simulink model "ATRIAS_vnmc"  (R2015a)
settings: Solver=ode45  StartTime=0.0  StopTime=60  FixedStep=1e-3  MinStep=1e-6  RelTol=1e-3  AbsTol=1e-4
values from neighbouring files (symbols this model uses):
  initial_boom_yaw = initial_boom_yaw + delta_yaw0    [run_model.m]
  max_floor_diff = cost_fun_opts.max_floor_diff    [opt_cmaes.m]    (also in run_model.m; set_all_params_simple.m = 0)
  noise_on_off = cost_fun_opts.noise_on_off    [opt_cmaes.m]    (also in run_model.m; set_all_params_simple.m = 0)
  noise_seed = cost_fun_opts.noise_seed    [opt_cmaes.m]    (also in run_model.m; set_all_params_simple.m = 1)
  noise_variance = cost_fun_opts.noise_variance    [opt_cmaes.m]    (also in run_model.m; set_all_params_simple.m = 0.000174532925199)
  SEA_swing_ctrl_on_off = cost_fun_opts.SEA_swing_ctrl_on_off    [opt_cmaes.m]    (also in run_model.m; set_all_params_simple.m = 0)
  sim_t = simout.twalk    [run_model.m]
  steady_dist = cost_fun_opts.steady_dist    [opt_cmaes.m]    (also in run_model.m; set_all_params_simple.m = 10)
  ts_anim = 0.0333    [run_model.m]
undefined symbols (not defined in the file or in its folder): A1_notch_f1, A2_notch_f1, A_lpf_dtau, A_lpf_velocity, B1_lpf_dtau, B1_lpf_velocity, B1_notch_f1, B2_lpf_dtau, B2_lpf_velocity, B2_notch_f1, b_hmotor, b_leg_spring, b_rotor, base_color_d, boom_color_d, boom_mount_to_center_diagonal, breakaway_friction, c, c_jointstop, com_height_offset, contactThr, coulomb_friction, CtrlPar_theta0, D12_S, D12_T, d_com, ddx_max, ddy_max, delta_phi_max, delta_phi_max_buffer, delta_phi_max_dropoff, delta_phi_min, des_forward_velocity, DS_width, dtau_des_max, dtheta0_vmc, dx0_vmc, dy_max, eref, fblink_color_d, fcut_acceleration, floor_color_d, floor_tile_width, floor_zero_height, FmaxBFSH, FmaxGLU, FmaxHAM, FmaxHFL, FmaxRF, FmaxVAS, FPCtrlPar, friction_linear_zone, g, gain_nodes_sea_torque, gamma_stance_thr, gamma_swing_thr, hip_height, HIP_MTR_MAX_CONT_TORQUE, HIP_MTR_MAX_TORQUE, hshaft_color_d ... (+236)
libraries: sm_lib x280, nesl_utility x174, simulink x114, simulink_extras x58, fl_lib x16, mblibv1 x2, dspswit3 x2
(part 8 of 23)

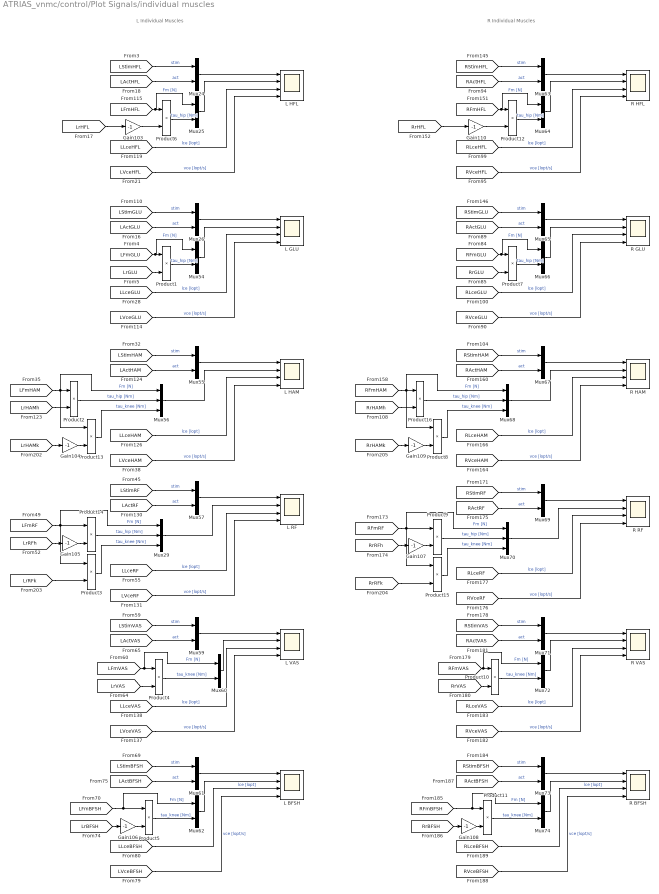
== system ATRIAS_vnmc/control/Plot Signals/individual muscles ==
  note: L Individual Muscles
  note: R Individual Muscles
  Gain{103..110} (8 alike) : Gain  Gain=-1
  L BFSH : Scope  NumInputPorts=4
      settings: ShowLegends=on  TimeRange=1  YMin=5.55112e-17~-50~0.65~-15  YMax=1~300~1~15  SaveName=ScopeData33
  L GLU : Scope  NumInputPorts=4
      settings: ShowLegends=on  TimeRange=1  YMin=0~0~0.4~-20  YMax=1~260.2739726027394~1~20  SaveName=ScopeData37
  L HAM : Scope  NumInputPorts=4
      settings: ShowLegends=on  TimeRange=1  YMin=0~-175.6756756756768~0.6000000000000001~-20  YMax=1~716.2162162162167~1~20  SaveName=ScopeData39
  L HFL : Scope  NumInputPorts=4
      settings: ShowLegends=on  TimeRange=1  YMin=0~-315.0684931506839~0.8~-20  YMax=1~424.6575342465767~1.4~20  SaveName=ScopeData41
  L RF : Scope  NumInputPorts=4
      settings: ShowLegends=on  TimeRange=1  YMin=0~-119.8630136986303~0.7000000000000001~-20  YMax=1~147.2602739726026~1~20  SaveName=ScopeData44
  L VAS : Scope  NumInputPorts=4
      settings: ShowLegends=on  TimeRange=2.5  YMin=0~0~0.5~-20  YMax=1~6000~1.5~20  SaveName=ScopeData47
  Mux{24..26,54..55,57,59..67,69,71..74} (20 alike) : Mux  Inputs=2
  Mux{29,56,68,70} (4 alike) : Mux  Inputs=3
  Product{1..16} (16 alike) : Product  RndMeth=Zero
  R BFSH : Scope  NumInputPorts=4
      settings: ShowLegends=on  TimeRange=1.6  YMin=130~-300~-5~-5  YMax=200~300~5~5  SaveName=ScopeData58
  R GLU : Scope  NumInputPorts=4
      settings: ShowLegends=on  TimeRange=1.6  YMin=130~-300~-5~-5  YMax=200~300~5~5  SaveName=ScopeData60
  R HAM : Scope  NumInputPorts=4
      settings: ShowLegends=on  TimeRange=1.6  YMin=130~-300~-5~-5  YMax=200~300~5~5  SaveName=ScopeData62
  R HFL : Scope  NumInputPorts=4
      settings: ShowLegends=on  TimeRange=1.6  YMin=130~-300~-5~-5  YMax=200~300~5~5  SaveName=ScopeData64
  R RF : Scope  NumInputPorts=4
      settings: ShowLegends=on  TimeRange=1.6  YMin=130~-300~-5~-5  YMax=200~300~5~5  SaveName=ScopeData67
  R VAS : Scope  NumInputPorts=4
      settings: ShowLegends=on  TimeRange=1.6  YMin=130~-300~-5~-5  YMax=200~300~5~5  SaveName=ScopeData70
  wires:
  [LStimHFL] -> Mux24/1  "stim"
  [LFmHFL] -> Mux25/1, Product6/1  "Fm [N]"
  [LrHFL] -> Gain103/1
  Product6/1 -> Mux25/2  "tau_hip [Nm]"
  [LActHFL] -> Mux24/2  "act"
  Mux24/1 -> L HFL/1
  Mux25/1 -> L HFL/2
  [LLceHFL] -> L HFL/3  "lce [lopt]"
  [LVceHFL] -> L HFL/4  "vce [lopt/s]"
  [LStimGLU] -> Mux26/1  "stim"
  [LFmGLU] -> Mux54/1, Product1/1  "Fm [N]"
  [LrGLU] -> Product1/2
  Product1/1 -> Mux54/2  "tau_hip [Nm]"
  [LActGLU] -> Mux26/2  "act"
  Mux26/1 -> L GLU/1
  Mux54/1 -> L GLU/2
  [LLceGLU] -> L GLU/3  "lce [lopt]"
  [LVceGLU] -> L GLU/4  "vce [lopt/s]"
  [LStimHAM] -> Mux55/1  "stim"
  [LFmHAM] -> Product2/1, Product13/1, Mux56/1  "Fm [N]"
  [LrHAMh] -> Product2/2
  Product2/1 -> Mux56/2  "tau_hip [Nm]"
  [LActHAM] -> Mux55/2  "act"
  Mux55/1 -> L HAM/1
  Mux56/1 -> L HAM/2
  [LLceHAM] -> L HAM/3  "lce [lopt]"
  [LVceHAM] -> L HAM/4  "vce [lopt/s]"
  [LStimRF] -> Mux57/1  "stim"
  [LActRF] -> Mux57/2  "act"
  Mux57/1 -> L RF/1
  [LLceRF] -> L RF/3  "lce [lopt]"
  [LVceRF] -> L RF/4  "vce [lopt/s]"
  [LStimVAS] -> Mux59/1  "stim"
  [LFmVAS] -> Product4/1, Mux60/1  "Fm [N]"
  Product4/1 -> Mux60/2  "tau_knee [Nm]"
  [LActVAS] -> Mux59/2  "act"
  Mux59/1 -> L VAS/1
  Mux60/1 -> L VAS/2
  [LLceVAS] -> L VAS/3  "lce [lopt]"
  [LVceVAS] -> L VAS/4  "vce [lopt/s]"
  [LStimBFSH] -> Mux61/1  "stim"
  [LFmBFSH] -> Mux62/1, Product5/1  "Fm [N]"
  [LrBFSH] -> Gain106/1
  Product5/1 -> Mux62/2  "tau_knee [Nm]"
  [LActBFSH] -> Mux61/2  "act"
  Mux61/1 -> L BFSH/1
  Mux62/1 -> L BFSH/2
  [LLceBFSH] -> L BFSH/3  "lce [lopt]"
  [LVceBFSH] -> L BFSH/4  "vce [lopt/s]"
  Gain103/1 -> Product6/2
  [LrHAMk] -> Gain104/1
  Product13/1 -> Mux56/3  "tau_knee [Nm]"
  [LFmRF] -> Product14/1, Product3/1, Mux29/1  "Fm [N]"
  [LrRFh] -> Gain105/1
  Product14/1 -> Mux29/2  "tau_hip [Nm]"
  [LrRFk] -> Product3/2
  Product3/1 -> Mux29/3  "tau_knee [Nm]"
  Gain105/1 -> Product14/2
  Mux29/1 -> L RF/2
  [LrVAS] -> Product4/2
  Gain106/1 -> Product5/2
  Gain104/1 -> Product13/2
  [RStimHFL] -> Mux63/1  "stim"
  [RFmHFL] -> Mux64/1, Product12/1  "Fm [N]"
  [RrHFL] -> Gain110/1
  Product12/1 -> Mux64/2  "tau_hip [Nm]"
  [RActHFL] -> Mux63/2  "act"
  Mux63/1 -> R HFL/1
  Mux64/1 -> R HFL/2
  [RLceHFL] -> R HFL/3  "lce [lopt]"
  [RVceHFL] -> R HFL/4  "vce [lopt/s]"
  [RStimGLU] -> Mux65/1  "stim"
  [RFmGLU] -> Mux66/1, Product7/1  "Fm [N]"
  [RrGLU] -> Product7/2
  Product7/1 -> Mux66/2  "tau_hip [Nm]"
  [RActGLU] -> Mux65/2  "act"
  Mux65/1 -> R GLU/1
  Mux66/1 -> R GLU/2
  [RLceGLU] -> R GLU/3  "lce [lopt]"
  [RVceGLU] -> R GLU/4  "vce [lopt/s]"
  [RStimHAM] -> Mux67/1  "stim"
  [RActHAM] -> Mux67/2  "act"
  Mux67/1 -> R HAM/1
  [RLceHAM] -> R HAM/3  "lce [lopt]"
  [RVceHAM] -> R HAM/4  "vce [lopt/s]"
  [RStimVAS] -> Mux71/1  "stim"
  [RFmVAS] -> Mux72/1, Product10/1  "Fm [N]"
  [RrVAS] -> Product10/2
  Product10/1 -> Mux72/2  "tau_knee [Nm]"
  [RActVAS] -> Mux71/2  "act"
  Mux71/1 -> R VAS/1
  Mux72/1 -> R VAS/2
  [RLceVAS] -> R VAS/3  "lce [lopt]"
  [RVceVAS] -> R VAS/4  "vce [lopt/s]"
  [RStimBFSH] -> Mux73/1  "stim"
  [RFmBFSH] -> Product11/1, Mux74/1  "Fm [N]"
  [RrBFSH] -> Gain108/1
  Product11/1 -> Mux74/2  "tau_knee [Nm]"
  [RActBFSH] -> Mux73/2  "act"
  Mux73/1 -> R BFSH/1
  Mux74/1 -> R BFSH/2
  [RLceBFSH] -> R BFSH/3  "lce [lopt]"
  [RVceBFSH] -> R BFSH/4  "vce [lopt/s]"
  [RStimRF] -> Mux69/1  "stim"
  [RActRF] -> Mux69/2  "act"
  Mux69/1 -> R RF/1
  [RLceRF] -> R RF/3  "lce [lopt]"
  [RVceRF] -> R RF/4  "vce [lopt/s]"
  [RFmRF] -> Product9/1, Product15/1, Mux70/1  "Fm [N]"
  [RrRFh] -> Gain107/1
  Product9/1 -> Mux70/2  "tau_hip [Nm]"
  [RrRFk] -> Product15/2
  Product15/1 -> Mux70/3  "tau_knee [Nm]"
  Gain107/1 -> Product9/2
  Mux70/1 -> R RF/2
  Gain108/1 -> Product11/2
  [RFmHAM] -> Product16/1, Product8/1, Mux68/1  "Fm [N]"
  [RrHAMh] -> Product16/2
  Product16/1 -> Mux68/2  "tau_hip [Nm]"
  Mux68/1 -> R HAM/2
  Product8/1 -> Mux68/3  "tau_knee [Nm]"
  Gain110/1 -> Product12/2
  [RrHAMk] -> Gain109/1
  Gain109/1 -> Product8/2

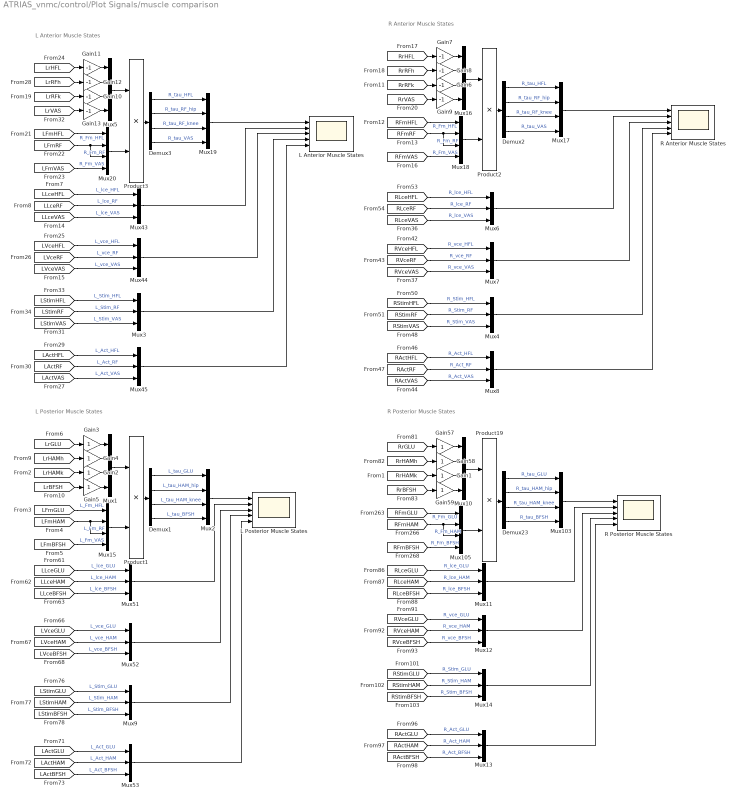
== system ATRIAS_vnmc/control/Plot Signals/muscle comparison ==
  note: R Anterior Muscle States
  note: L Anterior Muscle States
  note: L Posterior Muscle States
  note: R Posterior Muscle States
  Demux{1..3,23} (4 alike) : Demux
  Gain{1..5,57..59} (8 alike) : Gain
  Gain{6..13} (8 alike) : Gain  Gain=-1
  L Anterior Muscle States : Scope  NumInputPorts=5
      settings: ShowLegends=on  TimeRange=0.168  YMin=-500~0.7000000000000001~-15~0~0  YMax=-0~1.2~15~1~1  SaveName=ScopeData31
  L Posterior Muscle States : Scope  NumInputPorts=5
      settings: ShowLegends=on  TimeRange=0.168  YMin=0~0.6000000000000001~-15~0~0  YMax=200~1~15~1~1  SaveName=ScopeData43
  Mux{1..2,5,10,15..20,103,105} (12 alike) : Mux
  Mux{3..4,6..9,11..14,43..45,51..53} (16 alike) : Mux  Inputs=3
  Product{1..3,19} (4 alike) : Product
  R Anterior Muscle States : Scope  NumInputPorts=5
      settings: ShowLegends=on  TimeRange=60  YMin=-5000000000~-2500000000~-5000000000~-5~-5  YMax=4000000000~25000000000~4000000000~5~5  SaveName=ScopeData57
  R Posterior Muscle States : Scope  NumInputPorts=5
      settings: ShowLegends=on  TimeRange=0.4895299077760617  YMin=0~0.4~-15~-0.2~0  YMax=3500~1.6~5~1~0.8  SaveName=ScopeData66
  wires:
  [LLceHFL] -> Mux43/1  "L_lce_HFL"
  [LLceVAS] -> Mux43/3  "L_lce_VAS"
  [LLceRF] -> Mux43/2  "L_lce_RF"
  Mux43/1 -> L Anterior Muscle States/2
  [LVceRF] -> Mux44/2  "L_vce_RF"
  [LVceHFL] -> Mux44/1  "L_vce_HFL"
  Mux44/1 -> L Anterior Muscle States/3
  [LVceVAS] -> Mux44/3  "L_vce_VAS"
  [LActGLU] -> Mux53/1  "L_Act_GLU"
  [LLceHAM] -> Mux51/2  "L_lce_HAM"
  Mux45/1 -> L Anterior Muscle States/5
  [LActHFL] -> Mux45/1  "L_Act_HFL"
  [LActVAS] -> Mux45/3  "L_Act_VAS"
  Mux52/1 -> L Posterior Muscle States/3
  [LActRF] -> Mux45/2  "L_Act_RF"
  Mux51/1 -> L Posterior Muscle States/2
  [LActBFSH] -> Mux53/3  "L_Act_BFSH"
  [LLceBFSH] -> Mux51/3  "L_lce_BFSH"
  [LVceBFSH] -> Mux52/3  "L_vce_BFSH"
  [LLceGLU] -> Mux51/1  "L_lce_GLU"
  [LActHAM] -> Mux53/2  "L_Act_HAM"
  [LVceHAM] -> Mux52/2  "L_vce_HAM"
  Mux53/1 -> L Posterior Muscle States/5
  [LVceGLU] -> Mux52/1  "L_vce_GLU"
  Mux3/1 -> L Anterior Muscle States/4
  [LStimHFL] -> Mux3/1  "L_Stim_HFL"
  [LStimVAS] -> Mux3/3  "L_Stim_VAS"
  [LStimRF] -> Mux3/2  "L_Stim_RF"
  [RLceHFL] -> Mux6/1  "R_lce_HFL"
  [RLceVAS] -> Mux6/3  "R_lce_VAS"
  [RLceRF] -> Mux6/2  "R_lce_RF"
  Mux6/1 -> R Anterior Muscle States/2
  [RVceRF] -> Mux7/2  "R_vce_RF"
  [RVceHFL] -> Mux7/1  "R_vce_HFL"
  Mux7/1 -> R Anterior Muscle States/3
  [RVceVAS] -> Mux7/3  "R_vce_VAS"
  Mux8/1 -> R Anterior Muscle States/5
  [RActHFL] -> Mux8/1  "R_Act_HFL"
  [RActVAS] -> Mux8/3  "R_Act_VAS"
  [RActRF] -> Mux8/2  "R_Act_RF"
  Mux4/1 -> R Anterior Muscle States/4
  [RStimHFL] -> Mux4/1  "R_Stim_HFL"
  [RStimVAS] -> Mux4/3  "R_Stim_VAS"
  [RStimRF] -> Mux4/2  "R_Stim_RF"
  [LStimGLU] -> Mux9/1  "L_Stim_GLU"
  [LStimBFSH] -> Mux9/3  "L_Stim_BFSH"
  [LStimHAM] -> Mux9/2  "L_Stim_HAM"
  Mux9/1 -> L Posterior Muscle States/4
  [RActGLU] -> Mux13/1  "R_Act_GLU"
  [RLceHAM] -> Mux11/2  "R_lce_HAM"
  Mux12/1 -> R Posterior Muscle States/3
  Mux11/1 -> R Posterior Muscle States/2
  [RActBFSH] -> Mux13/3  "R_Act_BFSH"
  [RLceBFSH] -> Mux11/3  "R_lce_BFSH"
  [RVceBFSH] -> Mux12/3  "R_vce_BFSH"
  [RLceGLU] -> Mux11/1  "R_lce_GLU"
  [RActHAM] -> Mux13/2  "R_Act_HAM"
  [RVceHAM] -> Mux12/2  "R_vce_HAM"
  Mux13/1 -> R Posterior Muscle States/5
  [RVceGLU] -> Mux12/1  "R_vce_GLU"
  [RStimGLU] -> Mux14/1  "R_Stim_GLU"
  [RStimBFSH] -> Mux14/3  "R_Stim_BFSH"
  [RStimHAM] -> Mux14/2  "R_Stim_HAM"
  Mux14/1 -> R Posterior Muscle States/4
  [RFmBFSH] -> Mux105/4  "R_Fm_BFSH"
  [RFmHAM] -> Mux105/3, Mux105/2  "R_Fm_HAM"
  [RFmGLU] -> Mux105/1  "R_Fm_GLU"
  [RrBFSH] -> Gain59/1
  [RrHAMh] -> Gain58/1
  [RrGLU] -> Gain57/1
  Gain57/1 -> Mux10/1
  Gain58/1 -> Mux10/2
  Gain59/1 -> Mux10/4
  Mux10/1 -> Product19/1
  Mux105/1 -> Product19/2
  Demux23/2 -> Mux103/2  "R_tau_HAM_hip"
  Demux23/1 -> Mux103/1  "R_tau_GLU"
  Demux23/3 -> Mux103/3  "R_tau_HAM_knee"
  Product19/1 -> Demux23/1
  Mux103/1 -> R Posterior Muscle States/1
  [RrHAMk] -> Gain1/1
  Gain1/1 -> Mux10/3
  Demux23/4 -> Mux103/4  "R_tau_BFSH"
  [LFmBFSH] -> Mux15/4  "L_Fm_VAS"
  [LFmHAM] -> Mux15/3, Mux15/2  "L_Fm_RF"
  [LFmGLU] -> Mux15/1  "L_Fm_HFL"
  [LrBFSH] -> Gain5/1
  [LrHAMh] -> Gain4/1
  [LrGLU] -> Gain3/1
  Gain3/1 -> Mux1/1
  Gain4/1 -> Mux1/2
  Gain5/1 -> Mux1/4
  Mux1/1 -> Product1/1
  Mux15/1 -> Product1/2
  Demux1/2 -> Mux2/2  "L_tau_HAM_hip"
  Demux1/1 -> Mux2/1  "L_tau_GLU"
  Demux1/3 -> Mux2/3  "L_tau_HAM_knee"
  Product1/1 -> Demux1/1
  Mux2/1 -> L Posterior Muscle States/1
  [LrHAMk] -> Gain2/1
  Gain2/1 -> Mux1/3
  Demux1/4 -> Mux2/4  "L_tau_BFSH"
  [RFmVAS] -> Mux18/4  "R_Fm_VAS"
  [RFmRF] -> Mux18/3, Mux18/2  "R_Fm_RF"
  [RFmHFL] -> Mux18/1  "R_Fm_HFL"
  [RrVAS] -> Gain9/1
  [RrRFh] -> Gain8/1
  [RrHFL] -> Gain7/1
  Gain7/1 -> Mux16/1
  Gain8/1 -> Mux16/2
  Gain9/1 -> Mux16/4
  Mux16/1 -> Product2/1
  Mux18/1 -> Product2/2
  Demux2/2 -> Mux17/2  "R_tau_RF_hip"
  Demux2/1 -> Mux17/1  "R_tau_HFL"
  Demux2/3 -> Mux17/3  "R_tau_RF_knee"
  Product2/1 -> Demux2/1
  Mux17/1 -> R Anterior Muscle States/1
  [RrRFk] -> Gain6/1
  Gain6/1 -> Mux16/3
  Demux2/4 -> Mux17/4  "R_tau_VAS"
  [LFmVAS] -> Mux20/4  "R_Fm_VAS"
  [LFmRF] -> Mux20/3, Mux20/2  "R_Fm_RF"
  [LFmHFL] -> Mux20/1  "R_Fm_HFL"
  [LrVAS] -> Gain13/1
  [LrRFh] -> Gain12/1
  [LrHFL] -> Gain11/1
  Gain11/1 -> Mux5/1
  Gain12/1 -> Mux5/2
  Gain13/1 -> Mux5/4
  Mux5/1 -> Product3/1
  Mux20/1 -> Product3/2
  Demux3/2 -> Mux19/2  "R_tau_RF_hip"
  Demux3/1 -> Mux19/1  "R_tau_HFL"
  Demux3/3 -> Mux19/3  "R_tau_RF_knee"
  Product3/1 -> Demux3/1
  Mux19/1 -> L Anterior Muscle States/1
  [LrRFk] -> Gain10/1
  Gain10/1 -> Mux5/3
  Demux3/4 -> Mux19/4  "R_tau_VAS"

== system ATRIAS_vnmc/control/Plot Signals/muscle etc ==
  note: Muscle Moment Arms
  note: Muscle Lengths
  MTU Lengths : Scope  NumInputPorts=4
      settings: ShowLegends=on  TimeRange=0.4895299077760617  YMin=0.15~0.1~0.1~0.2  YMax=0.4500000000000001~0.4~0.4500000000000001~0.5  SaveName=ScopeData49
  Moment Arms : Scope  NumInputPorts=4
      settings: ShowLegends=on  TimeRange=0.4895299077760617  YMin=0~0.02~-0.04~0.04  YMax=0.08~0.08~0.08~0.08  SaveName=ScopeData56
  Mux{15..18} (4 alike) : Mux  Inputs=3
  Mux{19..22} (4 alike) : Mux
  wires:
  Mux15/1 -> MTU Lengths/1
  [LLmtuHFL] -> Mux15/1  "L_Lmtu_HFL"
  [LLmtuVAS] -> Mux15/3  "L_Lmtu_VAS"
  [LLmtuRF] -> Mux15/2  "L_Lmtu_RF"
  Mux16/1 -> MTU Lengths/2
  [RLmtuHFL] -> Mux16/1  "R_Lmtu_HFL"
  [RLmtuVAS] -> Mux16/3  "R_Lmtu_VAS"
  [RLmtuRF] -> Mux16/2  "R_Lmtu_RF"
  [LLmtuGLU] -> Mux17/1  "L_Lmtu_GLU"
  [LLmtuBFSH] -> Mux17/3  "L_Lmtu_BFSH"
  [LLmtuHAM] -> Mux17/2  "L_Lmtu_HAM"
  Mux17/1 -> MTU Lengths/3
  [RLmtuGLU] -> Mux18/1  "R_Lmtu_GLU"
  [RLmtuBFSH] -> Mux18/3  "R_Lmtu_BFSH"
  [RLmtuHAM] -> Mux18/2  "R_Lmtu_HAM"
  Mux18/1 -> MTU Lengths/4
  Mux19/1 -> Moment Arms/1
  [LrHFL] -> Mux19/1  "L_r_HFL"
  [LrVAS] -> Mux19/4  "L_r_VAS"
  [LrRFh] -> Mux19/2  "L_r_RF"
  [LrGLU] -> Mux21/1  "L_r_GLU"
  [LrBFSH] -> Mux21/4  "L_r_BFSH"
  [LrHAMh] -> Mux21/2  "L_r_HAM_h"
  Mux21/1 -> Moment Arms/3
  [LrRFk] -> Mux19/3  "L_r_RF_k"
  Mux20/1 -> Moment Arms/2
  [RrHFL] -> Mux20/1  "R_r_HFL"
  [RrVAS] -> Mux20/4  "R_r_VAS"
  [RrRFh] -> Mux20/2  "R_r_RF"
  [RrRFk] -> Mux20/3  "R_r_RF_k"
  [LrHAMk] -> Mux21/3  "L_r_HAM_k"
  [RrGLU] -> Mux22/1  "R_r_GLU"
  [RrBFSH] -> Mux22/4  "R_r_BFSH"
  [RrHAMh] -> Mux22/2  "R_r_HAM_h"
  Mux22/1 -> Moment Arms/4
  [RrHAMk] -> Mux22/3  "R_r_HAM_k"

== system ATRIAS_vnmc/control/Plot Signals/stims ==
  note: L Stimulation Modules
  note: R Stimulation Modules
  note: Swing Phases
  Demux10 : Demux  Outputs=7
  Demux{6,8,11..12,14,17} (6 alike) : Demux  Outputs=8
  Demux13 : Demux  Outputs=9
  Demux15 : Demux  Outputs=5
  Demux16 : Demux  Outputs=7
  Demux18 : Demux
  Demux19 : Demux
  Demux7 : Demux  Outputs=9
  Demux9 : Demux  Outputs=5
  L BFSH Stim Modules : Scope  NumInputPorts=8
      settings: ShowLegends=on  TimeRange=1.6  YMin=130~-300~-5~-5~-5~-5~-5~-5  YMax=200~300~5~5~5~5~5~5  SaveName=ScopeData35
  L GLU Stim Modules : Scope  NumInputPorts=9
      settings: ShowLegends=on  TimeRange=1.6  YMin=130~-300~-5~-5~-5~-5~-5~-5~-5  YMax=200~300~5~5~5~5~5~5~5  SaveName=ScopeData38
  L HAM Stim Modules : Scope  NumInputPorts=8
      settings: ShowLegends=on  TimeRange=1.6  YMin=130~-300~-5~-5~-5~-5~-5~-5  YMax=200~300~5~5~5~5~5~5  SaveName=ScopeData40
  L HFL Stim Modules : Scope  NumInputPorts=8
      settings: ShowLegends=on  TimeRange=1.6  YMin=130~-300~-5~-5~-5~-5~-5~-5  YMax=200~300~5~5~5~5~5~5  SaveName=ScopeData42
  L RF Stim Modules : Scope  NumInputPorts=5
      settings: ShowLegends=on  TimeRange=1.6  YMin=130~-300~-5~-5~-5  YMax=200~300~5~5~5  SaveName=ScopeData45
  L Swing Phases : Scope  NumInputPorts=4
      settings: ShowLegends=on  TimeRange=1.6  YMin=-0.1~-0.1~-5~-5  YMax=1.1~1.1~5~5  SaveName=ScopeData46
  L VAS Stim Modules : Scope  NumInputPorts=7
      settings: ShowLegends=on  TimeRange=1.6  YMin=130~-300~-5~-5~-5~-5~-5  YMax=200~300~5~5~5~5~5  SaveName=ScopeData48
  LModsBFSH : Selector  InputPortWidth=35  Indices=[6 12 17 28 30 32]
  LModsBFSH1 : Selector  InputPortWidth=35  Indices=[6 12 17 28 30 32]
  LModsGLU : Selector  InputPortWidth=35  Indices=[2 8 13 19 22 27 34]
  LModsGLU1 : Selector  InputPortWidth=35  Indices=[2 8 13 19 22 27 34]
  LModsHAM : Selector  InputPortWidth=35  Indices=[3 9 15 20 23 31]
  LModsHAM1 : Selector  InputPortWidth=35  Indices=[3 9 15 20 23 31]
  LModsHFL : Selector  InputPortWidth=35  Indices=[1 7 18 21 26 33]
  LModsHFL1 : Selector  InputPortWidth=35  Indices=[1 7 18 21 26 33]
  LModsRF : Selector  InputPortWidth=35  Indices=[4 10 29]
  LModsRF1 : Selector  InputPortWidth=35  Indices=[4 10 29]
  LModsVAS : Selector  InputPortWidth=35  Indices=[5 11 14 16 35]
  LModsVAS1 : Selector  InputPortWidth=35  Indices=[5 11 14 16 35]
  Mux{30..31,46..49,75..80} (12 alike) : Mux  Inputs=3
  R BFSH Stim Modules : Scope  NumInputPorts=8
      settings: ShowLegends=on  TimeRange=1.6  YMin=130~-300~-5~-5~-5~-5~-5~-5  YMax=200~300~5~5~5~5~5~5  SaveName=ScopeData59
  R GLU Stim Modules : Scope  NumInputPorts=9
      settings: ShowLegends=on  TimeRange=1.6  YMin=130~-300~-5~-5~-5~-5~-5~-5~-5  YMax=200~300~5~5~5~5~5~5~5  SaveName=ScopeData61
  R HAM Stim Modules : Scope  NumInputPorts=8
      settings: ShowLegends=on  TimeRange=1.6  YMin=130~-300~-5~-5~-5~-5~-5~-5  YMax=200~300~5~5~5~5~5~5  SaveName=ScopeData63
  R HFL Stim Modules : Scope  NumInputPorts=8
      settings: ShowLegends=on  TimeRange=1.6  YMin=130~-300~-5~-5~-5~-5~-5~-5  YMax=200~300~5~5~5~5~5~5  SaveName=ScopeData65
  R RF Stim Modules : Scope  NumInputPorts=5
      settings: ShowLegends=on  TimeRange=1.6  YMin=130~-300~-5~-5~-5  YMax=200~300~5~5~5  SaveName=ScopeData68
  R Swing Phases : Scope  NumInputPorts=4
      settings: ShowLegends=on  TimeRange=1.6  YMin=130~-300~-5~-5  YMax=200~300~5~5  SaveName=ScopeData69
  R VAS Stim Modules : Scope  NumInputPorts=7
      settings: ShowLegends=on  TimeRange=1.6  YMin=130~-300~-5~-5~-5~-5~-5  YMax=200~300~5~5~5~5~5  SaveName=ScopeData71
  wires:
  Demux6/3 -> L HFL Stim Modules/3  "M0_Sw"
  [LAct] -> LModsHFL/1
  Demux6/1 -> L HFL Stim Modules/1  "Total"
  Demux6/2 -> L HFL Stim Modules/2  "M0_St"
  Demux6/4 -> L HFL Stim Modules/4  "M3"
  Demux6/5 -> L HFL Stim Modules/5  "M4"
  Demux6/6 -> L HFL Stim Modules/6  "M6"
  Demux7/3 -> L GLU Stim Modules/3  "M0_Sw"
  Demux7/1 -> L GLU Stim Modules/1  "Total"
  Demux7/2 -> L GLU Stim Modules/2  "M0_St"
  Demux7/4 -> L GLU Stim Modules/4  "M1"
  Demux7/5 -> L GLU Stim Modules/5  "M3"
  Demux7/6 -> L GLU Stim Modules/6  "M4"
  Demux7/7 -> L GLU Stim Modules/7  "M6"
  Demux8/3 -> L HAM Stim Modules/3  "M0_Sw"
  Demux8/1 -> L HAM Stim Modules/1  "Total"
  Demux8/2 -> L HAM Stim Modules/2  "M0_St"
  Demux8/4 -> L HAM Stim Modules/4  "M2"
  Demux8/5 -> L HAM Stim Modules/5  "M3"
  Demux8/6 -> L HAM Stim Modules/6  "M4"
  Demux9/3 -> L RF Stim Modules/3  "M0_St"
  Demux9/2 -> L RF Stim Modules/2  "M0_St"
  Demux9/1 -> L RF Stim Modules/1  "Total"
  Demux16/3 -> L VAS Stim Modules/3  "M0_Sw"
  Demux16/1 -> L VAS Stim Modules/1  "Total"
  Demux16/2 -> L VAS Stim Modules/2  "M0_St"
  Demux16/4 -> L VAS Stim Modules/4  "M1"
  Demux16/5 -> L VAS Stim Modules/5  "M2"
  Demux17/3 -> L BFSH Stim Modules/3  "M0_Sw"
  Demux17/1 -> L BFSH Stim Modules/1  "Total"
  Demux17/2 -> L BFSH Stim Modules/2  "M0_St"
  Demux17/4 -> L BFSH Stim Modules/4  "M2"
  Demux17/5 -> L BFSH Stim Modules/5  "M7"
  Demux17/6 -> L BFSH Stim Modules/6  "M8"
  Mux30/1 -> Demux6/1
  [LStance] -> Mux30/3
  Demux6/7 -> L HFL Stim Modules/7  "M10"
  [LStimHFL] -> Mux30/1
  LModsHFL/1 -> Mux30/2
  Demux6/8 -> L HFL Stim Modules/8  "Stance"
  Demux7/9 -> L GLU Stim Modules/9  "Stance"
  Demux7/8 -> L GLU Stim Modules/8  "M10"
  [LAct] -> LModsGLU/1
  LModsGLU/1 -> Mux31/2
  [LStimGLU] -> Mux31/1
  [LStance] -> Mux31/3
  Mux31/1 -> Demux7/1
  [LAct] -> LModsHAM/1
  LModsHAM/1 -> Mux46/2
  [LStimHAM] -> Mux46/1
  [LStance] -> Mux46/3
  Mux46/1 -> Demux8/1
  Demux8/7 -> L HAM Stim Modules/7  "M9"
  Demux8/8 -> L HAM Stim Modules/8  "Stance"
  [LAct] -> LModsRF/1
  LModsRF/1 -> Mux47/2
  [LStimRF] -> Mux47/1
  [LStance] -> Mux47/3
  Mux47/1 -> Demux9/1
  Demux9/4 -> L RF Stim Modules/4  "M8"
  Demux9/5 -> L RF Stim Modules/5  "Stance"
  Demux16/6 -> L VAS Stim Modules/6  "M10"
  Demux16/7 -> L VAS Stim Modules/7  "Stance"
  [LAct] -> LModsVAS/1
  LModsVAS/1 -> Mux48/2
  [LStimVAS] -> Mux48/1
  [LStance] -> Mux48/3
  Mux48/1 -> Demux16/1
  [LAct] -> LModsBFSH/1
  LModsBFSH/1 -> Mux49/2
  [LStimBFSH] -> Mux49/1
  [LStance] -> Mux49/3
  Mux49/1 -> Demux17/1
  Demux17/7 -> L BFSH Stim Modules/7  "M9"
  Demux17/8 -> L BFSH Stim Modules/8  "Stance"
  Demux12/3 -> R HFL Stim Modules/3  "M0_Sw"
  [RAct] -> LModsHFL1/1
  Demux12/1 -> R HFL Stim Modules/1  "Total"
  Demux12/2 -> R HFL Stim Modules/2  "M0_St"
  Demux12/4 -> R HFL Stim Modules/4  "M3"
  Demux12/5 -> R HFL Stim Modules/5  "M4"
  Demux12/6 -> R HFL Stim Modules/6  "M6"
  Demux13/3 -> R GLU Stim Modules/3  "M0_Sw"
  Demux13/1 -> R GLU Stim Modules/1  "Total"
  Demux13/2 -> R GLU Stim Modules/2  "M0_St"
  Demux13/4 -> R GLU Stim Modules/4  "M1"
  Demux13/5 -> R GLU Stim Modules/5  "M3"
  Demux13/6 -> R GLU Stim Modules/6  "M4"
  Demux13/7 -> R GLU Stim Modules/7  "M6"
  Demux14/3 -> R HAM Stim Modules/3  "M0_Sw"
  Demux14/1 -> R HAM Stim Modules/1  "Total"
  Demux14/2 -> R HAM Stim Modules/2  "M0_St"
  Demux14/4 -> R HAM Stim Modules/4  "M2"
  Demux14/5 -> R HAM Stim Modules/5  "M3"
  Demux14/6 -> R HAM Stim Modules/6  "M4"
  Demux15/3 -> R RF Stim Modules/3  "M0_St"
  Demux15/2 -> R RF Stim Modules/2  "M0_St"
  Demux15/1 -> R RF Stim Modules/1  "Total"
  Demux10/3 -> R VAS Stim Modules/3  "M0_Sw"
  Demux10/1 -> R VAS Stim Modules/1  "Total"
  Demux10/2 -> R VAS Stim Modules/2  "M0_St"
  Demux10/4 -> R VAS Stim Modules/4  "M1"
  Demux10/5 -> R VAS Stim Modules/5  "M2"
  Demux11/3 -> R BFSH Stim Modules/3  "M0_Sw"
  Demux11/1 -> R BFSH Stim Modules/1  "Total"
  Demux11/2 -> R BFSH Stim Modules/2  "M0_St"
  Demux11/4 -> R BFSH Stim Modules/4  "M2"
  Demux11/5 -> R BFSH Stim Modules/5  "M7"
  Demux11/6 -> R BFSH Stim Modules/6  "M8"
  Mux75/1 -> Demux12/1
  [RStance] -> Mux75/3
  Demux12/7 -> R HFL Stim Modules/7  "M10"
  [RStimHFL] -> Mux75/1
  LModsHFL1/1 -> Mux75/2
  Demux12/8 -> R HFL Stim Modules/8  "Stance"
  Demux13/9 -> R GLU Stim Modules/9  "Stance"
  Demux13/8 -> R GLU Stim Modules/8  "M10"
  [RAct] -> LModsGLU1/1
  LModsGLU1/1 -> Mux76/2
  [RStimGLU] -> Mux76/1
  [RStance] -> Mux76/3
  Mux76/1 -> Demux13/1
  [RAct] -> LModsHAM1/1
  LModsHAM1/1 -> Mux77/2
  [RStimHAM] -> Mux77/1
  [RStance] -> Mux77/3
  Mux77/1 -> Demux14/1
  Demux14/7 -> R HAM Stim Modules/7  "M9"
  Demux14/8 -> R HAM Stim Modules/8  "Stance"
  [RAct] -> LModsRF1/1
  LModsRF1/1 -> Mux78/2
  [RStimRF] -> Mux78/1
  [RStance] -> Mux78/3
  Mux78/1 -> Demux15/1
  Demux15/4 -> R RF Stim Modules/4  "M8"
  Demux15/5 -> R RF Stim Modules/5  "Stance"
  Demux10/6 -> R VAS Stim Modules/6  "M10"
  Demux10/7 -> R VAS Stim Modules/7  "Stance"
  [RAct] -> LModsVAS1/1
  LModsVAS1/1 -> Mux79/2
  [RStimVAS] -> Mux79/1
  [RStance] -> Mux79/3
  Mux79/1 -> Demux10/1
  [RAct] -> LModsBFSH1/1
  LModsBFSH1/1 -> Mux80/2
  [RStimBFSH] -> Mux80/1
  [RStance] -> Mux80/3
  Mux80/1 -> Demux11/1
  Demux11/7 -> R BFSH Stim Modules/7  "M9"
  Demux11/8 -> R BFSH Stim Modules/8  "Stance"
  Demux18/3 -> L Swing Phases/3  "L_M9"
  [LSwingPhase] -> Demux18/1
  Demux18/1 -> L Swing Phases/1  "L_M7"
  Demux18/2 -> L Swing Phases/2  "L_M8"
  Demux18/4 -> L Swing Phases/4  "L_M10"
  Demux19/3 -> R Swing Phases/3  "R_M9"
  [RSwingPhase] -> Demux19/1
  Demux19/1 -> R Swing Phases/1  "R_M7"
  Demux19/2 -> R Swing Phases/2  "R_M8"
  Demux19/4 -> R Swing Phases/4  "R_M10"

== system ATRIAS_vnmc/control/Plot Signals/virtual joint torques ==
  Hip/Knee/Virtual Limit Torques : Scope  NumInputPorts=2
      settings: ShowLegends=on  TimeRange=0.4  YMin=0~-200  YMax=350~150  SaveName=ScopeData30
  Mux : Mux
  Mux1 : Mux
  wires:
  [LM12] -> Mux/1  "LM12"
  [RM12] -> Mux/2  "RM12"
  [LKneeStop] -> Mux/3  "LM12_stop"
  [RKneeStop] -> Mux/4  "RM12_stop"
  Mux/1 -> Hip/Knee/Virtual Limit Torques/1
  [LM23] -> Mux1/1  "LM23"
  [RM23] -> Mux1/2  "RM23"
  [LHipStop] -> Mux1/3  "LM23_stop"
  [RHipStop] -> Mux1/4  "RM23_stop"
  Mux1/1 -> Hip/Knee/Virtual Limit Torques/2

== system ATRIAS_vnmc/control/Robot-to-NMM Interface/L Leg Load ==
  tau_F [Nm] : Inport
  tau_B [Nm] : Inport  Port=2
  splay [rad] : Inport  Port=3
  Calculate Leg Load : Fcn  Expr=1/(2*l_seg*sin(u(3)/2))*u(1)-1/(2*l_seg*sin(u(3)/2))*u(2)
  Mux : Mux  Inputs=3
  Positive Values only : Saturate  UpperLimit=Inf  LowerLimit=0
  Leg Load [N] : Outport
  wires:
  tau_F [Nm]/1 -> Mux/1
  tau_B [Nm]/1 -> Mux/2
  splay [rad]/1 -> Mux/3
  Mux/1 -> Calculate Leg Load/1
  Positive Values only/1 -> Leg Load [N]/1
  Calculate Leg Load/1 -> Positive Values only/1

== system ATRIAS_vnmc/control/Robot-to-NMM Interface/R Leg Geometry f(l_seg, l_v, v12_max) ==
  qBack [rad] : Inport
  qFront [rad] : Inport  Port=2
  dqBack [rad/s] : Inport  Port=3
  dqFront [rad/s] : Inport  Port=4
  Constant : Constant  Value=pi/2
  Constant1 : Constant  Value=l_seg/l_v
  Divide : Product  Inputs=**/
  Fcn : Fcn  Expr=(1-u(3))/2*u(1) + (1+u(3))/2*u(2)
  Fcn1 : Fcn  Expr=-u(3)*u(1) + u(3)*u(2)
  Gain : Gain  Gain=0.5
  Gain1 : Gain  Gain=0.5
  Gain2 : Gain  Gain=l_seg/l_v
  Gain3 : Gain  Gain=2
  Gain4 : Gain  Gain=0.5
  Mux : Mux  Inputs=3
  Sum : Sum  Inputs=|+-
  Sum1 : Sum  Inputs=|+-
  Sum2 : Sum  Inputs=|++
  Sum3 : Sum  Inputs=|++
  Trigonometric Function : Trigonometry  Operator=cos
  Trigonometric Function1 : Trigonometry  Operator=asin
  Trigonometric Function2 : Trigonometry
  Trigonometric Function3 : Trigonometry  Operator=cos
  "[0,sin(v12_max/2)]" : Saturate  UpperLimit=sin(v12_max/2)  LowerLimit=0
  "[0,v12_max]" : Saturate  UpperLimit=v12_max  LowerLimit=0
  "[min_splay_angle/2, inf]" : Saturate  UpperLimit=inf  LowerLimit=min_splay_angle/2
  virtual knee angle [rad] : Outport
  virtual knee velocity [rad/s] : Outport  Port=2
  virtual hip angle [rad] : Outport  Port=3
  virtual hip velocity [rad/s] : Outport  Port=4
  k : Outport  Port=5
  wires:
  Sum/1 -> Gain/1
  qBack [rad]/1 -> [qB]
  qFront [rad]/1 -> [qF]
  dqBack [rad/s]/1 -> [dqB]
  dqFront [rad/s]/1 -> [dqF]
  [qF] -> Sum3/2, Sum/2
  [qB] -> Sum/1, Sum3/1
  Gain/1 -> Trigonometric Function/1, "[min_splay_angle/2, inf]"/1
  [phiK] -> Gain1/1
  Sum1/1 -> Sum2/1
  Constant/1 -> Sum1/2
  Gain1/1 -> Trigonometric Function3/1, Sum2/2
  Sum2/1 -> [phiH]
  Trigonometric Function/1 -> Gain2/1
  Gain2/1 -> "[0,sin(v12_max/2)]"/1
  "[0,sin(v12_max/2)]"/1 -> Trigonometric Function1/1
  Trigonometric Function1/1 -> "[0,v12_max]"/1
  "[0,v12_max]"/1 -> Gain3/1
  Gain3/1 -> [phiK]
  [phiK] -> virtual knee angle [rad]/1
  [phiH] -> virtual hip angle [rad]/1
  Trigonometric Function2/1 -> Divide/2
  Constant1/1 -> Divide/1
  Trigonometric Function3/1 -> Divide/3
  Divide/1 -> k/1, Mux/3
  Mux/1 -> Fcn/1, Fcn1/1
  [dqF] -> Mux/2
  [dqB] -> Mux/1
  Fcn/1 -> virtual hip velocity [rad/s]/1
  Fcn1/1 -> virtual knee velocity [rad/s]/1
  Sum3/1 -> Gain4/1
  Gain4/1 -> Sum1/1
  "[min_splay_angle/2, inf]"/1 -> Trigonometric Function2/1

== system ATRIAS_vnmc/control/Robot-to-NMM Interface/R Leg Geometry f(l_seg, l_v, v12_max)1 ==
  qBack [rad] : Inport
  qFront [rad] : Inport  Port=2
  dqBack [rad/s] : Inport  Port=3
  dqFront [rad/s] : Inport  Port=4
  Constant : Constant  Value=pi/2
  Constant1 : Constant  Value=l_seg/l_v
  Divide : Product  Inputs=**/
  Fcn : Fcn  Expr=(1-u(3))/2*u(1) + (1+u(3))/2*u(2)
  Fcn1 : Fcn  Expr=-u(3)*u(1) + u(3)*u(2)
  Gain : Gain  Gain=0.5
  Gain1 : Gain  Gain=0.5
  Gain2 : Gain  Gain=l_seg/l_v
  Gain3 : Gain  Gain=2
  Gain4 : Gain  Gain=0.5
  Mux : Mux  Inputs=3
  Sum : Sum  Inputs=|+-
  Sum1 : Sum  Inputs=|+-
  Sum2 : Sum  Inputs=|++
  Sum3 : Sum  Inputs=|++
  Trigonometric Function : Trigonometry  Operator=cos
  Trigonometric Function1 : Trigonometry  Operator=asin
  Trigonometric Function2 : Trigonometry
  Trigonometric Function3 : Trigonometry  Operator=cos
  "[0,sin(v12_max/2)]" : Saturate  UpperLimit=sin(v12_max/2)  LowerLimit=0
  "[0,v12_max]" : Saturate  UpperLimit=v12_max  LowerLimit=0
  "[min_splay_angle/2, inf]" : Saturate  UpperLimit=inf  LowerLimit=min_splay_angle/2
  virtual knee angle [rad] : Outport
  virtual knee velocity [rad/s] : Outport  Port=2
  virtual hip angle [rad] : Outport  Port=3
  virtual hip velocity [rad/s] : Outport  Port=4
  k : Outport  Port=5
  wires:
  "[min_splay_angle/2, inf]"/1 -> Trigonometric Function2/1
  Gain4/1 -> Sum1/1
  Sum3/1 -> Gain4/1
  Fcn1/1 -> virtual knee velocity [rad/s]/1
  Fcn/1 -> virtual hip velocity [rad/s]/1
  [dqB] -> Mux/1
  [dqF] -> Mux/2
  Mux/1 -> Fcn1/1, Fcn/1
  Divide/1 -> Mux/3, k/1
  Trigonometric Function3/1 -> Divide/3
  Constant1/1 -> Divide/1
  Trigonometric Function2/1 -> Divide/2
  [phiH] -> virtual hip angle [rad]/1
  [phiK] -> virtual knee angle [rad]/1
  Gain3/1 -> [phiK]
  "[0,v12_max]"/1 -> Gain3/1
  Trigonometric Function1/1 -> "[0,v12_max]"/1
  "[0,sin(v12_max/2)]"/1 -> Trigonometric Function1/1
  Gain2/1 -> "[0,sin(v12_max/2)]"/1
  Trigonometric Function/1 -> Gain2/1
  Sum2/1 -> [phiH]
  Gain1/1 -> Sum2/2, Trigonometric Function3/1
  Constant/1 -> Sum1/2
  Sum1/1 -> Sum2/1
  [phiK] -> Gain1/1
  Gain/1 -> "[min_splay_angle/2, inf]"/1, Trigonometric Function/1
  [qB] -> Sum3/1, Sum/1
  [qF] -> Sum/2, Sum3/2
  dqFront [rad/s]/1 -> [dqF]
  dqBack [rad/s]/1 -> [dqB]
  qFront [rad]/1 -> [qF]
  qBack [rad]/1 -> [qB]
  Sum/1 -> Gain/1

== system ATRIAS_vnmc/control/Robot-to-NMM Interface/R Leg Load ==
  tau_F [Nm] : Inport
  tau_B [Nm] : Inport  Port=2
  splay [rad] : Inport  Port=3
  Calculate Leg Load : Fcn  Expr=1/(2*l_seg*sin(u(3)/2))*u(1)-1/(2*l_seg*sin(u(3)/2))*u(2)
  Mux : Mux  Inputs=3
  Positive Values only : Saturate  UpperLimit=Inf  LowerLimit=0
  Leg Load [N] : Outport
  wires:
  Calculate Leg Load/1 -> Positive Values only/1
  Positive Values only/1 -> Leg Load [N]/1
  Mux/1 -> Calculate Leg Load/1
  splay [rad]/1 -> Mux/3
  tau_B [Nm]/1 -> Mux/2
  tau_F [Nm]/1 -> Mux/1

== system ATRIAS_vnmc/control/SEA Ctrl/Activate SEA Control ==
  SEA Control Signal [Nm] x4 : Inport
  "SEA on/off [1/0] x4 " : Inport  Port=2
  Torque Signal [Nm] x4 : Inport  Port=3
  Demux : Demux
  Demux2 : Demux
  Demux3 : Demux
  Mux6 : Mux
  Switch{,1..3} (4 alike) : Switch  Criteria=u2 ~= 0
  Torque Command [Nm] x4 : Outport
  wires:
  Demux2/2 -> Switch1/3
  Demux2/1 -> Switch/3
  Demux/1 -> Switch/1
  Switch/1 -> Mux6/1
  Switch1/1 -> Mux6/2
  Switch3/1 -> Mux6/4
  Demux3/1 -> Switch/2
  Mux6/1 -> Torque Command [Nm] x4/1
  Demux3/3 -> Switch2/2
  Demux3/2 -> Switch1/2
  Demux/3 -> Switch2/1
  Switch2/1 -> Mux6/3
  Demux/4 -> Switch3/1
  Demux2/4 -> Switch3/3
  Demux3/4 -> Switch3/2
  Demux/2 -> Switch1/1
  Demux2/3 -> Switch2/3
  SEA Control Signal [Nm] x4/1 -> Demux/1
  "SEA on/off [1/0] x4 "/1 -> Demux3/1
  Torque Signal [Nm] x4/1 -> Demux2/1

== system ATRIAS_vnmc/control/SEA Ctrl/Antiresonance Compensation ==
  Torque : Inport
  Notch Filter (Flight) : DiscreteTransferFcn  Numerator=[K_notch_f1 K_notch_f1*A1_notch_f1 K_notch_f1*A2_notch_f1]  Denominator=[1 B1_notch_f1 B2_notch_f1]  SampleTime=sample_time
  Filtered Torque : Outport
  wires:
  Torque/1 -> Notch Filter (Flight)/1
  Notch Filter (Flight)/1 -> Filtered Torque/1

== system ATRIAS_vnmc/control/SEA Ctrl/SEA Controller (Torque) ==
  phi_load [rad] x4 : Inport
  phi_gear [rad] x4 : Inport  Port=2
  tau_des sagittal [Nm] x4 : Inport  Port=3
  dtau_des sagittal [Nm] x4 : Inport  Port=4
  dphi_load [rad/s] x4 : Inport  Port=5
  dphi_gear [rad/s] x4 : Inport  Port=6
  (L Back) SEA Components : Scope  NumInputPorts=4
      settings: ShowLegends=on  TimeRange=0.224  YMin=-10~-500~-600~-1  YMax=40~300~400~1  SaveName=ScopeData18
  (L Front) SEA Components : Scope  NumInputPorts=4
      settings: ShowLegends=on  TimeRange=0.224  YMin=-40~-200~-400~-1  YMax=10~300~300~1  SaveName=ScopeData19
  (R Back) SEA Components : Scope  NumInputPorts=4
      settings: ShowLegends=on  YMin=-500~-1500~-500~0  YMax=100~1500~500~1  SaveName=ScopeData16
  (R Front) SEA Components : Scope  NumInputPorts=4
      settings: ShowLegends=on  TimeRange=0.224  YMin=0~-400~-200~0  YMax=150~800~600~1  SaveName=ScopeData17
  Abs : Abs
  Antiresonance Compensation : Subsystem
  D gain ramp : Lookup_n-D  NumberOfTableDimensions=1  BreakpointsForDimension1=gain_nodes_sea_torque  Table=kd_sea_torque  InternalRulePriority=Speed  RndMeth=Simplest  InputSameDT=on
  Demux{,1..8} (9 alike) : Demux
  Friction Compensation : Subsystem
  Loaded Unloaded Switch : Subsystem
  Mux{,1..3,8..11} (8 alike) : Mux  Inputs=2
  Mux{4..7} (4 alike) : Mux
  P gain ramp : Lookup_n-D  NumberOfTableDimensions=1  BreakpointsForDimension1=gain_nodes_sea_torque  Table=kp_sea_torque  InternalRulePriority=Speed  RndMeth=Simplest  InputSameDT=on
  Product : Product  SampleTime=sample_time  RndMeth=Zero
  Product2 : Product  RndMeth=Zero
  Spring Stiffness : Gain  Gain=k_sea
  Spring Stiffness 1 : Gain  Gain=k_sea
  Sum1 : Sum  Inputs=-+|
  Sum10 : Sum  Inputs=|++
  Sum2 : Sum  Inputs=|+-
  Sum3 : Sum  Inputs=++|
  Sum5 : Sum  Inputs=|+-
  Sum6 : Sum  Inputs=-+|
  Sum7 : Sum  Inputs=+|+
  Torque Limiter (outside) 1 : Saturate  UpperLimit=max_sagittal_loaded_torque  LowerLimit=-max_sagittal_loaded_torque
      settings: AttributesFormatString=Hi: %<UpperLimit>\nLo: %<LowerLimit>
  Torque Limiter (outside) 2 : Saturate  Commented=on  UpperLimit=dtau_des_max  LowerLimit=-dtau_des_max
      settings: AttributesFormatString=Hi: %<UpperLimit>\nLo: %<LowerLimit>
  Torque Limiter (outside) 3 : Saturate  UpperLimit=max_sagittal_unloaded_torque  LowerLimit=-max_sagittal_unloaded_torque
      settings: AttributesFormatString=Hi: %<UpperLimit>\nLo: %<LowerLimit>
  Torque Threshold : simulink/Logic and Bit Operations/Compare To Constant  relop=>=  const=loaded_unloaded_torque_threshold  OutDataTypeStr=boolean
  filtered_derivative : Subsystem  Commented=on
  kd_gain1 : Gain  Description=xPCTag(1)=kd_sea_torque;  Commented=on  Gain=i_motor_reflected
  kd_gain3 : Gain  Description=xPCTag(1)=kd_sea_torque;  Commented=on  Gain=k_ff
  tau_cmd sagittal [Nm] x4 : Outport
  tau_measured [Nm] x4 : Outport  Port=2
  wires:
  Product2/1 -> Sum7/2, Demux3/1
  D gain ramp/1 -> Product2/1
  Sum2/1 -> Product2/2
  Sum5/1 -> Product/2
  dphi_gear [rad/s] x4/1 -> Friction Compensation/1(Motor Velocity [rad/s]), Sum6/2
  dphi_load [rad/s] x4/1 -> Sum6/1, filtered_derivative/1(x)
  Spring Stiffness 1/1 -> Sum2/2
  Sum6/1 -> Spring Stiffness 1/1
  tau_des sagittal [Nm] x4/1 -> Sum5/1, Demux/1, Sum3/1
  phi_gear [rad] x4/1 -> Sum1/2
  phi_load [rad] x4/1 -> Sum1/1
  Sum1/1 -> Spring Stiffness/1
  Spring Stiffness/1 -> Demux1/1, Sum5/2, Abs/1, tau_measured [Nm] x4/1
  Sum10/1 -> Antiresonance Compensation/1(Torque), Torque Limiter (outside) 1/1
  P gain ramp/1 -> Product/1
  Product/1 -> Sum7/1, Demux2/1
  Sum7/1 -> Sum3/2
  Torque Limiter (outside) 1/1 -> Demux5/1, Loaded Unloaded Switch/1(Loaded Signal)
  Torque Limiter (outside) 3/1 -> Demux6/1, Loaded Unloaded Switch/2(Unloaded Signal)
  Antiresonance Compensation/1(Filtered Torque) -> Torque Limiter (outside) 3/1
  Friction Compensation/1(Friction Compensation [Nm]) -> Demux4/1, Sum10/2
  Loaded Unloaded Switch/1(Signal) -> tau_cmd sagittal [Nm] x4/1
  Torque Threshold/1 -> Demux7/1, Loaded Unloaded Switch/3(Loaded/Unloaded [1/0] x4)
  Abs/1 -> Torque Threshold/1, D gain ramp/1, P gain ramp/1
  Sum3/1 -> Sum10/1
  kd_gain1/1 -> kd_gain3/1
  filtered_derivative/1(dx/dt) -> kd_gain1/1
  kd_gain3/1 -> Demux8/1
  Demux/1 -> Mux/1  "tau_des (feedforward) [Nm]"
  Demux1/1 -> Mux/2  "tau_meas [Nm]"
  Demux/2 -> Mux1/1  "tau_des (feedforward)  [Nm]"
  Demux/3 -> Mux2/1  "tau_des (feedforward)  [Nm]"
  Demux/4 -> Mux3/1  "tau_des (feedforward)  [Nm]"
  Demux1/2 -> Mux1/2  "tau_meas [Nm]"
  Demux1/3 -> Mux2/2  "tau_meas [Nm]"
  Demux1/4 -> Mux3/2  "tau_meas [Nm]"
  Mux/1 -> (R Back) SEA Components/1
  Demux2/1 -> Mux4/1  "Kp term[Nm]"
  Demux3/1 -> Mux4/2  "Kd term [Nm]"
  Demux4/1 -> Mux4/3  "friction compensation [Nm]"
  Demux2/2 -> Mux5/1  "Kp term[Nm]"
  Demux3/2 -> Mux5/2  "Kd term [Nm]"
  Demux4/2 -> Mux5/3  "friction compensation [Nm]"
  Demux2/3 -> Mux6/1  "Kp term[Nm]"
  Demux3/3 -> Mux6/2  "Kd term [Nm]"
  Demux4/3 -> Mux6/3  "friction compensation [Nm]"
  Demux2/4 -> Mux7/1  "Kp term[Nm]"
  Demux3/4 -> Mux7/2  "Kd term [Nm]"
  Demux4/4 -> Mux7/3  "friction compensation [Nm]"
  Demux5/1 -> Mux8/1  "loaded cmd [Nm]"
  Demux6/1 -> Mux8/2  "unloaded cmd [Nm]"
  Demux5/2 -> Mux9/1  "loaded cmd [Nm]"
  Demux6/2 -> Mux9/2  "unloaded cmd [Nm]"
  Demux5/3 -> Mux10/1  "loaded cmd [Nm]"
  Demux6/3 -> Mux10/2  "unloaded cmd [Nm]"
  Demux6/4 -> Mux11/2  "unloaded cmd [Nm]"
  Demux5/4 -> Mux11/1  "loaded cmd [Nm]"
  Mux4/1 -> (R Back) SEA Components/2
  Mux8/1 -> (R Back) SEA Components/3
  Demux7/1 -> (R Back) SEA Components/4  "loaded/unloaded [0/1]"
  Mux1/1 -> (R Front) SEA Components/1
  Mux5/1 -> (R Front) SEA Components/2
  Mux9/1 -> (R Front) SEA Components/3
  Demux7/2 -> (R Front) SEA Components/4  "loaded/unloaded [0/1]"
  Mux2/1 -> (L Back) SEA Components/1
  Mux6/1 -> (L Back) SEA Components/2
  Mux10/1 -> (L Back) SEA Components/3
  Demux7/3 -> (L Back) SEA Components/4  "loaded/unloaded [0/1]"
  Mux3/1 -> (L Front) SEA Components/1
  Mux7/1 -> (L Front) SEA Components/2
  Mux11/1 -> (L Front) SEA Components/3
  Demux7/4 -> (L Front) SEA Components/4  "loaded/unloaded [0/1]"
  Demux8/1 -> Mux4/4  "Kff term [Nm]"
  Demux8/2 -> Mux5/4  "Kff term [Nm]"
  Demux8/3 -> Mux6/4  "Kff term [Nm]"
  Demux8/4 -> Mux7/4  "Kff term [Nm]"
  dtau_des sagittal [Nm] x4/1 -> Sum2/1

== system ATRIAS_vnmc/control/Virtual Model Control/COM PD Law ==
  Clock : Clock
  Clock1 : Clock
  Clock2 : Clock  Commented=on
  Constant1 : Constant  Value=start_forward_velocity_time
  Constant10 : Constant  Value=y0_vmc_end
  Constant13 : Constant  Commented=on  Value=y0_vmc_end
  Constant15 : Constant  Value=kp_y_vmc
  Constant16 : Constant  Commented=on  Value=0
  Constant17 : Constant  Value=kd_y_vmc
  Constant18 : Constant  Value=theta0_vmc
  Constant19 : Constant  Value=kp_theta_vmc
  Constant2 : Constant  Value=des_forward_velocity
  Constant20 : Constant  Value=dtheta0_vmc
  Constant21 : Constant  Value=kd_theta_vmc
  Constant3 : Constant  Commented=on  Value=y0_transition_time
  Constant33 : Constant  Value=kp_x_vmc
  Constant34 : Constant  Commented=on  Value=dx0_vmc
  Constant35 : Constant  Value=kd_x_vmc
  Constant4 : Constant  Value=0
  Constant5 : Constant  Commented=on  Value=ddy_max
  Constant6 : Constant  Commented=on  Value=dy_max
  Constant7 : Constant  Commented=on  Value=0
  Constant8 : Constant  Commented=on  Value=y0_vmc_start
  Constant9 : Constant  Value=0
  Demux : Demux  Outputs=2
  Demux1 : Demux  Commented=on  Outputs=2
  Demux2 : Demux  Commented=on  Outputs=3
  Detect Change : simulink/Logic and Bit Operations/Detect Change  vinit=0  InputProcessing=Inherited  OutDataTypeStr=boolean
  Detect Change1 : simulink/Logic and Bit Operations/Detect Change  vinit=0  InputProcessing=Inherited  OutDataTypeStr=boolean
  Detect Change2 : simulink/Logic and Bit Operations/Detect Change  vinit=0  InputProcessing=Inherited  OutDataTypeStr=boolean
  From : From  Commented=on  GotoTag=start_forward  TagVisibility=global
  From2 : From  Commented=on  GotoTag=y_com  TagVisibility=global
  Hold Values : Subsystem
  Hold Values1 : Subsystem  Commented=on
  Integrator : Integrator  ExternalReset=rising  InitialConditionSource=external
  Logical Operator : Logic  Operator=OR  Inputs=3  AllPortsSameDT=off  OutDataTypeStr=boolean
  Min-time y_com trajectory : MATLAB Function  Commented=on  TreatAsAtomicUnit=on
  Mux : Mux  Inputs=2
  Mux1 : Mux  Commented=on  Inputs=2
  Mux2 : Mux  Commented=on  Inputs=3
  Mux3 : Mux  Commented=on  Inputs=3
  Product{6..9,26..27} (6 alike) : Product
  Relational Operator : RelationalOperator  Operator=>  OutDataTypeStr=boolean
  Sum{3,10,12,31} (4 alike) : Sum  Inputs=|++
  Sum{9,11,13..14,30,32} (6 alike) : Sum  Inputs=|+-
  Sum4 : Sum  Commented=on  Inputs=|+-
  Switch : Switch  Criteria=u2 > Threshold  Threshold=start_forward_velocity_time
  Switch1 : Switch  Commented=on  Criteria=u2 ~= 0
  Terminator : Terminator  Commented=on
  Terminator1 : Terminator
  ddtheta_max1 : Saturate  UpperLimit=ddx_max  LowerLimit=-ddx_max
  ddx_max : Saturate  UpperLimit=ddx_max  LowerLimit=-ddx_max
  ddy_max : Saturate  UpperLimit=ddx_max  LowerLimit=-ddx_max
  low-pass : TransferFcn  Denominator=[tau_start 1]
  tag scope: ddtheta_des=global, ddtheta_des_d_term=global, ddtheta_des_p_term=global, ddx_des=global, ddx_des_d_term=global, ddx_des_p_term=global, ddy_des=global, ddy_des_d_term=global, ddy_des_p_term=global, dx_com_des=global, dy_com_des=global, start_forward=global, x_com_des=global, y_com_des=global
  wires:
  Sum30/1 -> Product26/2
  Product26/1 -> [ddx_des_p_term], Sum31/1
  Switch/1 -> low-pass/1
  Constant35/1 -> Product27/1
  Sum32/1 -> Product27/2
  Product27/1 -> [ddx_des_d_term], Sum31/2
  Sum31/1 -> ddx_max/1
  Constant33/1 -> Product26/1
  [x_com] -> Sum30/2
  [dx_com] -> Sum32/2
  Constant13/1 -> Min-time y_com trajectory/3(l_leg_final)
  Sum9/1 -> Product6/2
  Product6/1 -> [ddy_des_p_term], Sum10/1
  Constant16/1 -> Mux3/2
  Constant17/1 -> Product7/1
  Sum11/1 -> Product7/2
  Product7/1 -> [ddy_des_d_term], Sum10/2
  Sum10/1 -> Sum3/1
  Constant15/1 -> Product6/1
  [y_com] -> Sum9/2
  [dy_com] -> Sum11/2
  Constant18/1 -> Sum14/1
  Sum14/1 -> Product8/2
  Product8/1 -> [ddtheta_des_p_term], Sum12/1
  Constant20/1 -> Sum13/1
  Constant21/1 -> Product9/1
  Sum13/1 -> Product9/2
  Product9/1 -> [ddtheta_des_d_term], Sum12/2
  Sum12/1 -> ddtheta_max1/1
  Constant19/1 -> Product8/1
  [theta] -> Sum14/2
  [dtheta] -> Sum13/2
  Hold Values/1(out) -> Demux/1
  [Rstance_VMC] -> Detect Change/1
  [Lstance_VMC] -> Detect Change1/1
  Detect Change1/1 -> Logical Operator/2
  Detect Change/1 -> Logical Operator/1
  Logical Operator/1 -> Integrator/2, Hold Values/Trigger
  [x_com] -> Mux/1
  Mux/1 -> Hold Values/1(in)
  Clock/1 -> Mux/2
  Demux/1 -> Integrator/3
  Integrator/1 -> [x_com_des], Sum30/1
  Constant2/1 -> Switch/1
  Constant4/1 -> Switch/3
  Clock1/1 -> Relational Operator/1
  Detect Change2/1 -> Logical Operator/3
  ddx_max/1 -> [ddx_des]
  ddy_max/1 -> [ddy_des]
  ddtheta_max1/1 -> [ddtheta_des]
  low-pass/1 -> [dx_com_des], Sum32/1, Integrator/1
  Constant1/1 -> Relational Operator/2
  Sum3/1 -> ddy_max/1
  Hold Values1/1(out) -> Demux1/1
  Relational Operator/1 -> Switch/2, [start_forward]
  From2/1 -> Mux1/2
  Mux1/1 -> Hold Values1/1(in)
  Clock2/1 -> Sum4/1, Mux1/1
  Demux1/1 -> Sum4/2
  Sum4/1 -> Min-time y_com trajectory/1(t)  "delta t"
  Constant5/1 -> Min-time y_com trajectory/6(max_leg_acceleration)
  Constant6/1 -> Min-time y_com trajectory/5(max_leg_velocity)
  Constant3/1 -> Min-time y_com trajectory/4(t_trajectory)
  Demux1/2 -> Min-time y_com trajectory/2(l_leg_initial)
  Min-time y_com trajectory/1(l_leg) -> Mux2/1
  Min-time y_com trajectory/2(dl_leg) -> Mux2/2
  Min-time y_com trajectory/3(ddl_leg) -> Mux2/3
  Mux2/1 -> Switch1/1
  Mux3/1 -> Switch1/3
  From/1 -> Switch1/2
  Constant7/1 -> Mux3/3
  Switch1/1 -> Demux2/1
  Constant8/1 -> Mux3/1
  Constant10/1 -> [y_com_des], Sum9/1
  Constant9/1 -> [dy_com_des], Sum11/1
  Demux2/3 -> Terminator/1  "ff"
  Demux/2 -> Terminator1/1
  [start_forward] -> Detect Change2/1

== system ATRIAS_vnmc/control/Virtual Model Control/Double Support Geometry ==
  note: Starting Stance Geometry
  note: First-step Geometry
  Constant1 : Constant  Value=DS_width
  Constant2 : Constant  Value=hip_height
  Constant3 : Constant  Value=step_width
  Constant4 : Constant  Value=vmc_alpha_tgt
  Constant5 : Constant  Value=pi/2
  Constant6 : Constant  Value=2*pi
  Constant7 : Constant  Value=hip_height
  DS geometry : MATLAB Function  TreatAsAtomicUnit=on
  Demux : Demux  Outputs=2
  Divide : Product  Inputs=*/
  Mux : Mux  Inputs=2
  Terminator : Terminator
  Terminator1 : Terminator
  Trigonometric Function : Trigonometry
  convert to take-off angle : Sum  Inputs=+-
  gamma_tgt : Sum
  tag scope: gamma_max=global, gamma_min=global, leg_length_max=global, leg_length_min=global
  wires:
  Constant3/1 -> DS geometry/1(step_width)
  Constant1/1 -> DS geometry/2(DS_width)
  Constant2/1 -> DS geometry/3(height)
  DS geometry/1(L_min) -> [leg_length_min]
  DS geometry/3(gamma_min) -> [gamma_min]
  Constant4/1 -> Trigonometric Function/1, gamma_tgt/1
  Constant5/1 -> gamma_tgt/2
  gamma_tgt/1 -> convert to take-off angle/2
  Constant6/1 -> convert to take-off angle/1
  convert to take-off angle/1 -> Mux/2  "gamma_max"
  Constant7/1 -> Divide/1
  Trigonometric Function/1 -> Divide/2
  Divide/1 -> Mux/1  "L_max"
  Mux/1 -> Demux/1
  Demux/1 -> [leg_length_max]
  Demux/2 -> [gamma_max]
  DS geometry/2(L_max) -> Terminator/1
  DS geometry/4(gamma_max) -> Terminator1/1

== system ATRIAS_vnmc/control/Virtual Model Control/Estimate COM Position ==
  Constant{5,7,9..10,12} (5 alike) : Constant  Value=l_boom
  Constant11 : Constant  Value=com_height_offset
  Constant{4,6,8,14,23} (5 alike) : Constant  Value=boom_mount_to_center_diagonal
  Gain : Gain  Gain=-1
  Product1 : Product  Inputs=3
  Product2 : Product  Inputs=3
  Product3 : Product  Inputs=4
  Product4 : Product
  Product5 : Product  Inputs=3
  Sum{2..6,8} (6 alike) : Sum  Inputs=|++
  Sum7 : Sum  Inputs=|+-
  Trigonometric Function : Trigonometry  Operator=cos
  Trigonometric Function1 : Trigonometry  Operator=cos
  Trigonometric Function2 : Trigonometry
  Trigonometric Function3 : Trigonometry
  Trigonometric Function4 : Trigonometry  Operator=cos
  tag scope: dx_com=global, dy_com=global, x_com=global, y_com=global
  wires:
  [yaw] -> Product1/1
  Sum2/1 -> Product1/3
  Constant5/1 -> Sum2/1
  Constant4/1 -> Sum2/2
  Trigonometric Function/1 -> Product1/2
  [roll] -> Trigonometric Function/1
  Product1/1 -> [x_com]  "x"
  [dyaw] -> Product2/1
  Sum3/1 -> Product2/3
  Constant7/1 -> Sum3/1
  Constant6/1 -> Sum3/2
  Trigonometric Function1/1 -> Product2/2
  [roll] -> Trigonometric Function1/1
  Product2/1 -> Sum4/1  "x"
  [yaw] -> Product3/3
  Sum5/1 -> Product3/4
  Constant9/1 -> Sum5/1
  Constant8/1 -> Sum5/2
  Trigonometric Function2/1 -> Gain/1
  [roll] -> Trigonometric Function2/1
  Product3/1 -> Sum4/2
  Gain/1 -> Product3/2
  [droll] -> Product3/1
  Sum4/1 -> [dx_com]
  Sum6/1 -> Product4/2
  Constant10/1 -> Sum6/1
  Constant23/1 -> Sum6/2
  Trigonometric Function3/1 -> Product4/1
  [roll] -> Trigonometric Function3/1
  Product4/1 -> Sum7/1
  Constant11/1 -> Sum7/2
  Sum7/1 -> [y_com]
  Sum8/1 -> Product5/3
  Constant12/1 -> Sum8/1
  Constant14/1 -> Sum8/2
  Trigonometric Function4/1 -> Product5/2
  [roll] -> Trigonometric Function4/1
  Product5/1 -> [dy_com]
  [droll] -> Product5/1
